simulink model "roadIntersection"  (R2017a)
settings: Solver=VariableStepAuto  StartTime=0  StopTime=40  MaxStep=0.05  RelTol=1e-3
model workspace (MAT data in the model file):
  MCOS : class17 (value not decoded)
  MCOS : class17 (value not decoded)
  MCOS : class17 (value not decoded)
  MCOS : class17 (value not decoded)
  MCOS : class17 (value not decoded)
  MCOS : class17 (value not decoded)
  MCOS : class17 (value not decoded)
  MCOS : class17 (value not decoded)
values from neighbouring files (symbols this model uses):
  D = getSimulinkBlockHandle('experiment/Orientation')    [configModel.m]
  m = rt.find('-isa','Simulink.BlockDiagram','-and','Name',mdl)    [configModel.m]
  MIN_SAFE_DIST = 1    [simulation.m]    (also in stateflowSim.m)
  V = getSimulinkBlockHandle('experiment/Velocity')    [configModel.m]
  WORLD_SIZE = 8    [simulation.m]    (also in stateflowSim.m)
  X = getSimulinkBlockHandle('experiment/Position')    [configModel.m]
undefined symbols (not defined in the file or in its folder): DrivingState, n, Stateflow
libraries: libraries x28
(part 2 of 2)

== stateflow chart roadIntersection/Conservative ==
  state Left
    en:
    [pf,df] = prepareLeft(this);
    S(this) = DrivingState.LeftTurn;
    TURN.data(1) = -1.5;
    send(TURN);
    state Normal
      state Clear
      state Check
      (default) -> Left.Normal.Clear
      Left.Normal.Clear -> Check : [isCloseToCheck(this) && ...
          | hasOncomingCar(this)]
          | {send(BRAKE);}
      Check -> Left.Normal.Clear : [~hasOncomingCar(this)]
          | {send(GAS);}
    state WAIT
    Left.Normal -> Left.WAIT : [detectPedestrian]
    Left.WAIT -> Left.Normal : [~hasPedestrian(this,...
        | MIN_SAFE_DIST,...
        | 0.5*MIN_SAFE_DIST)]
        | {send(GAS);}
    (default) -> Left.Normal
  note: Helper Funcs
  note: Left Turn
  note: Right Turn
  note: Perception
  state Right
    en:
    [pf,df] = prepareRight(this);
    TURN.data(1) = 0.5;
    send(TURN);
    S(this) = DrivingState.RightTurn;
    state Normal
    state WAIT
    Right.Normal -> Right.WAIT : [detectPedestrian]
    Right.WAIT -> Right.Normal : [~hasPedestrian(this,...
        | MIN_SAFE_DIST,...
        | 0.5*MIN_SAFE_DIST)]
        | {send(GAS);}
    (default) -> Right.Normal
  state Straight
    en:
    S(this) = DrivingState.Straight;
    state HasFrontCar
      en:
      idx = frontCarIndex(this);
      state FollowBehind
        en:
        [dxnorm, dvnorm] = frontCarInfo(this,idx);
        du:
        [dxnorm, dvnorm] = frontCarInfo(this,idx);
        state Safe
          en:
          if dvnorm < 0
          disp('BRAKE');
          BRAKE.data = ...
          [norm(V(:,idx));A_MAX];
          send(BRAKE);
          else
          disp('GAS');
          GAS.data = ...
          [norm(V(:,idx));A_MAX]
          send(GAS);
          end
        state Dangerous
        Straight.HasFrontCar.FollowBehind.Safe -> Straight.HasFrontCar.FollowBehind.Dangerous : [dxnorm < 1.6 * MIN_SAFE_DIST]
            | {BRAKE.data = ...
            | [0.5*norm(V(:,idx));A_MAX];
            | send(BRAKE);}
        Straight.HasFrontCar.FollowBehind.Dangerous -> Straight.HasFrontCar.FollowBehind.Safe : [dxnorm > 2*MIN_SAFE_DIST]
        (junction 192) -> Straight.HasFrontCar.FollowBehind.Dangerous : {BRAKE.data = ...
            | [0;A_MAX];
            | send(BRAKE);}
        (junction 185) -> Straight.HasFrontCar.FollowBehind.Safe [order 1] : [dxnorm > 2 * MIN_SAFE_DIST]
        (default) -> (junction 185)
        (junction 185) -> (junction 192) [order 2]
    state FreeDriving
    (default) -> Straight.HasFrontCar [order 1] : [hasFrontCar(this)]
    (default) -> (junction 218) [order 2]
    Straight.HasFrontCar -> (junction 218) : [frontCarHasLeft(this)]
    (junction 218) -> Straight.FreeDriving : {GAS.data = [V_MAX;A_MAX];
        | send(GAS);}
    Straight.FreeDriving -> Straight.HasFrontCar : [hasFrontCar(this)]
  state Start
    en:
    GAS.data=[0;0];
    BRAKE.data=[0;0];
    TURN.data=[0;0];
    BACK.data=[0;0];
  state res = detectPedestrian [function]
    (default) -> (junction 241) : {res = false;}
    (junction 241) -> (junction 252) [order 1] : PEDES
    (junction 252) -> (junction 254) : {TRASH.data = PEDES.data;
        | forward(PEDES,TRASH);}
    (junction 254) -> (junction 241) : {res = true;}
    (junction 241) -> (junction 243) [order 2]
  state WAIT
  state RoadIntersection
    state FreeDriving
      state Normal
        state Green
          en:
          GAS.data = [V_MAX;A_MAX];
          send(GAS);
        state Stop
        state RushToPass
          en:
          GAS.data=...
          [V_MAX;A_MAX];
          send(GAS);
        (default) -> RoadIntersection.FreeDriving.Normal.Green [order 1] : [isGreen(this)]
        RoadIntersection.FreeDriving.Normal.Green -> (junction 211) : [isYellow(this)]
        RoadIntersection.FreeDriving.Normal.Stop -> RoadIntersection.FreeDriving.Normal.Green : [isGreen(this)]
        (junction 211) -> RoadIntersection.FreeDriving.Normal.Stop [order 1] : [norm(V(:,this)) == 0]
        (default) -> (junction 211) [order 2]
        (junction 211) -> (junction 209) [order 2]
        (junction 209) -> RushToPass [order 2]
        (junction 209) -> RoadIntersection.FreeDriving.Normal.Stop [order 1] : [isStoppable(this,inter)]
            | {BRAKE.data = ...
            | [0;requiredBrake(this,inter)];
            | send(BRAKE);}
      state Right
        state Clear
          state Green
            en:
            if norm(V(:,this)) < 1
            GAS.data = [1;A_MAX];
            send(GAS);
            elseif norm(V(:,this)) > 1
            BRAKE.data = [1;A_MAX];
            send(BRAKE);
            end
          state Stop
            en:
            if norm(V(:,this)) > 0
            BRAKE.data = ...
            [0;requiredBrake(this,inter)];
            send(BRAKE);
            end
          (default) -> RoadIntersection.FreeDriving.Right.Clear.Green [order 1] : [isGreen(this)]
          RoadIntersection.FreeDriving.Right.Clear.Stop -> RoadIntersection.FreeDriving.Right.Clear.Green : [isGreen(this)]
          RoadIntersection.FreeDriving.Right.Clear.Green -> RoadIntersection.FreeDriving.Right.Clear.Stop : [isYellow(this)]
          (default) -> RoadIntersection.FreeDriving.Right.Clear.Stop [order 2]
        state Wait
          en:
          BRAKE.data = ...
          [0;requiredBrake(this,inter)];
          send(BRAKE);
        (default) -> RoadIntersection.FreeDriving.Right.Clear [order 2]
        Wait -> RoadIntersection.FreeDriving.Right.Clear : [~pedCrossAtRight(inter)]
        RoadIntersection.FreeDriving.Right.Clear -> Wait : [pedCrossAtRight(inter)]
        (default) -> Wait [order 1] : [pedCrossAtRight(inter)]
      (default) -> RoadIntersection.FreeDriving.Normal [order 1] : [decision ~= Decision.Right]
      (default) -> RoadIntersection.FreeDriving.Right [order 2]
    state HasFrontCar
      en:
      idx = frontCarIndex(this);
      front = closestObj(this,X(:,idx),inter);
      du:
      front = closestObj(this,X(:,idx),inter);
      state FollowBehind
        en:
        [dxnorm, dvnorm] = frontCarInfo(this,idx);
        du:
        [dxnorm, dvnorm] = frontCarInfo(this,idx);
        state Safe
          en:
          if dvnorm < 0
          BRAKE.data(1) = ...
          norm(V(:,idx));
          send(BRAKE);
          else
          GAS.data(1) = ...
          norm(V(:,idx));
          send(GAS);
          end
        state Dangerous
        RoadIntersection.HasFrontCar.FollowBehind.Safe -> RoadIntersection.HasFrontCar.FollowBehind.Dangerous : [dxnorm < 1.4*MIN_SAFE_DIST]
            | {BRAKE.data = ...
            | [0.5*norm(V(:,this));A_MAX];
            | send(BRAKE);}
        RoadIntersection.HasFrontCar.FollowBehind.Dangerous -> RoadIntersection.HasFrontCar.FollowBehind.Safe : [dxnorm > 1.5*MIN_SAFE_DIST]
        (junction 200) -> RoadIntersection.HasFrontCar.FollowBehind.Dangerous : {BRAKE.data = ...
            | [0;A_MAX];
            | send(BRAKE);}
        (junction 198) -> RoadIntersection.HasFrontCar.FollowBehind.Safe [order 1] : [dxnorm > 1.5*MIN_SAFE_DIST]
        (default) -> (junction 198)
        (junction 198) -> (junction 200) [order 2]
      state Stop
        en:
        if norm(V(:,this)) > 0
        BRAKE.data = ...
        [0;requiredBrake(this,front)];
        send(BRAKE);
        end
      (default) -> RoadIntersection.HasFrontCar.FollowBehind [order 1] : [isGreen(this)]
      (default) -> (junction 182) [order 2]
      RoadIntersection.HasFrontCar.FollowBehind -> (junction 182) : [isYellow(this)]
      (junction 182) -> RoadIntersection.HasFrontCar.Stop
      RoadIntersection.HasFrontCar.Stop -> RoadIntersection.HasFrontCar.FollowBehind : [isGreen(this)]
    (default) -> RoadIntersection.FreeDriving
    RoadIntersection.FreeDriving -> RoadIntersection.HasFrontCar : [hasFrontCar(this)]
    RoadIntersection.HasFrontCar -> RoadIntersection.FreeDriving : [frontCarHasLeft(this) ||...
        | isequal(front,inter)]
  Left -> (junction 317) : [finishTurn(this,pf)]
      | {send(BACK);
      | inter = ...
      | resumeFromLeft(this,df);}
  (junction 76) -> Left
  (junction 317) -> (junction 318)
  (junction 48) -> (junction 76) [order 2]
  (junction 48) -> Right [order 1] : [decision == Decision.Right]
  (junction 44) -> (junction 48) [order 2]
  Right -> Straight : [finishTurn(this,pf)]
      | {send(BACK);
      | inter = ...
      | resumeFromRight(this,df);}
  (default) -> Start
  (junction 318) -> Straight
  Start -> Straight
  (junction 44) -> Straight [order 1] : [decision == Decision.Straight]
  RoadIntersection -> (junction 44) [order 1] : [passStopLine(this)]
  Straight -> RoadIntersection : [isCloseToInter(this)]
  WAIT -> RoadIntersection : [~hasPedestrian(this,...
      | MIN_SAFE_DIST,...
      | 0.5*MIN_SAFE_DIST)]
  RoadIntersection -> WAIT [order 2] : [detectPedestrian]
  data: dxfr function_output; self function_input; index function_input; dvfr function_output; self function_input; res function_output; self function_input uint8 size=1; p function_output; d function_output; self function_input; res function_output; lSafeDist function_input; sSafeDist function_input; self function_input uint8 size=1; d function_input; newInter function_output; self function_input uint8 size=1; d function_input; newInter function_output; self function_input; res function_output; self function_input; p function_input; res function_output; self function_input uint8 size=1; p function_output; d function_output; res function_output; currInter function_input; self function_input; res function_output; self function_input; idx function_output; self function_input; res function_output; self function_input; res function_output; self function_input; obj1 function_input; res function_output; obj2 function_input; self function_input; res function_output; self function_input; pos function_input; res function_output; dxnorm local; dvnorm local; idx local; self function_input; pos function_input; res function_output; self function_input; res function_output; res function_output; self function_input; res function_output; dxnorm local; dvnorm local; idx local; front local; inter local =[0.5; -1]; X data_store_memory; V data_store_memory; D data_store_memory; this local uint8 size=1 =uint8(2); GAS output; BRAKE output; MIN_SAFE_DIST parameter; light data_store_memory; WORLD_SIZE parameter; decision local Enum: Decision =Decision.Right; TURN output; pf local; df local; BACK output; V_MAX constant double =2.5; A_MAX constant double =2.5; P data_store_memory; PEDES input; TRASH local size=2; S data_store_memory
  function [dxfr,dvfr] = frontCarInfo(self,index):
    | function [dxfr,dvfr] = frontCarInfo(self,index)
    |  
    | x = X(:,self);
    | v = V(:,self);
    | d = D(:,self);
    | 
    | xfront = X(:,index);
    | vfront = V(:,index);
    | 
    | range = 2 * WORLD_SIZE;
    | 
    | dxfr = mod((dot(xfront - x, d)+range), range);
    | dvfr = dot(vfront-v, d);
  function res = hasOncomingCar(self):
    | function res = hasOncomingCar(self)
    |  
    | res = true;
    | 
    | xself = X(:, self);
    | xall = X;
    | [~,indx]=ismember(xself', xall', 'rows');
    | xall(:,indx) = [100; 100];
    | 
    | xmin = 0;
    | xmax = 0;
    | ymin = 0;
    | ymax = 0;
    | 
    | if isequal(inter, [0.5; -1])
    |     % region 1
    |     xmin = -1;
    |     ymax = 2.5;
    | elseif isequal(inter, [1; 0.5])
    |     % region 2
    |     ymin = -1;
    |     xmin = -2.5;
    | elseif isequal(inter, [-0.5; 1])
    |     % region 3 
    |     xmax = 1;
    |     ymin = -2.5;
    | elseif isequal(inter, [-1; -0.5])
    |     % region 4
    |     xmax = 2.5;
    |     ymax = 1;
    | else
    |     error('checkOncomingLane error');
    | end
    | 
    | xall = xall(:, (xall(1,:) >= xmin));
    | if ~isempty(xall)
    |     xall = xall(:, (xall(1,:) <= xmax));
    | else
    |     res = false;
    |     return;
    | end
    | if ~isempty(xall)
    |     xall = xall(:, (xall(2,:) >= ymin));
    | else
    |     res = false;
    |     return;
    | end
    | if ~isempty(xall)
    |     xall = xall(:, (xall(2,:) <= ymax));
    | else
    |     res = false;
    |     return;
    | end
  function [p, d] = prepareRight(self):
    | function [p, d] = prepareRight(self)
    | 
    | d0 = D(:,self);
    | p = [0; 0];
    | d = [0; 0];
    | 
    | if isequal(d0, [1; 0])
    |     p = [-0.5; -1];
    |     d = [0; -1];
    | elseif isequal(d0, [-1; 0])
    |     p = [0.5; 1];
    |     d = [0; 1];
    | elseif isequal(d0, [0; 1])
    |     p = [1; -0.5];
    |     d = [1; 0];
    | elseif isequal(d0, [0; -1])
    |     p = [-1; 0.5];
    |     d = [-1; 0];
    | else
    |     error('Unknown orientation');
    | end
  function res = hasPedestrian(self, lSafeDist, sSafeDist):
    | function res = hasPedestrian(self, lSafeDist, sSafeDist)
    | 
    | if ~any(P ~= -1)
    |     res = false;
    |     return;
    | end
    | 
    | FARAWAY = 100;
    | 
    | pi = [-1 1 1 1; -1 -1 1 1];
    | dp = [2 0 -2 0; 0 2 0 -2];
    | 
    | dx_norm = ones(4, 1) * FARAWAY;
    | x = X(:,self);
    | d = D(:,self);
    | 
    | offset = 0;
    | if S(self) == DrivingState.RightTurn
    |     offset = 0.5236;
    | elseif S(self) == DrivingState.LeftTurn
    |     offset = -0.5236;
    |     lSafeDist = 1.5*lSafeDist;
    | end
    | 
    | for k=1:length(P)
    |     
    |     if P(k) ~= -1
    |         p = pi(:,k) + dp(:,k) * P(k); 
    |         dx = p - x;
    |         
    |         check = dot(dx, d); 
    |         if check > 0
    |             
    |             dx_theta = atan2(dx(2), dx(1));
    |             d_theta = atan2(d(2), d(1));
    |             delta = d_theta - dx_theta;
    |         
    |             if delta > 3.1416 
    |                 delta = delta - 6.2832;
    |             elseif delta < -3.1416
    |                 delta = delta + 6.2832;
    |             end
    |             dx_norm(k) = norm(dx);
    |             
    |             % check nomalized angle lower than 30 degree
    |             if abs(delta-offset) > 0.5236 && (dx_norm(k) >= sSafeDist)
    |                 dx_norm(k) = FARAWAY;
    |             end
    |         end
    |         
    | %         check = dot(dx, d);
    | %         if check > 0
    | %             dx_norm(k) = norm(dx);
    | %             theta = acos(check/dx_norm(k));
    | %             if rad2deg(theta) > 30 && (dx_norm(k) >= sSafeDist)
    | %                 dx_norm(k) = FARAWAY;
    | %             end
    | %         end
    |     end
    | end
    | 
    | res = any(dx_norm <= 1 * lSafeDist);
  function newInter = resumeFromLeft(self, d):
    | function newInter = resumeFromLeft(self, d)
    | 
    | x = X(:,self);
    | 
    | if isequal(d, [1; 0])
    |     x = [1; -0.5];
    |     newInter = [-1; -0.5];
    | elseif isequal(d, [-1; 0])
    |     x = [-1; 0.5];
    |     newInter = [1; 0.5];
    | elseif isequal(d, [0; 1])
    |     x = [0.5; 1];
    |     newInter = [0.5; -1];
    | elseif isequal(d, [0; -1])
    |     x = [-0.5; -1];
    |     newInter = [-0.5; 1];
    | else
    |     error('Unknown orientation');
    | end
    | 
    | v = V(:,self);
    | 
    | X(:,self) = x;
    | V(:,self) = d * norm(v);
    | D(:,self) = d;
  function newInter = resumeFromRight(self, d):
    | function newInter = resumeFromRight(self, d)
    | 
    | x = X(:,self);
    | 
    | if isequal(d, [0; -1])
    |     x = [-0.5; -1];
    |     newInter = [-0.5; 1];
    | elseif isequal(d, [0; 1])
    |     x = [0.5; 1];
    |     newInter = [-0.5; -1];
    | elseif isequal(d, [1; 0])
    |     x = [1; -0.5];
    |     newInter = [-1; -0.5];
    | elseif isequal(d, [-1; 0])
    |     x = [-1; 0.5];
    |     newInter = [1; 0.5];
    | else
    |     error('Unknown orientation');
    | end
    | 
    | v = V(:,self);
    | 
    | X(:,self) = x;
    | V(:,self) = d * norm(v);
    | D(:,self) = d;
  function res = passStopLine(self):
    | function res = passStopLine(self)
    | 
    | x = X(:,self);
    | d = D(:,self);
    | 
    | dx_norm = dot(inter - x, d);
    | res = (dx_norm <= 0);
  function res = finishTurn(self, p):
    | function res = finishTurn(self, p)
    | 
    | x = X(:,self);
    | res = norm(x - p) <= 0.1;
  function [p, d] = prepareLeft(self):
    | function [p, d] = prepareLeft(self)
    | 
    | d0 = D(:,self);
    | p = [0; 0];
    | d = [0; 0];
    | 
    | if isequal(d0, [1; 0])
    |     p = [0.5; 1];
    |     d = [0; 1];
    | elseif isequal(d0, [-1; 0])
    |     p = [-0.5; -1];
    |     d = [0; -1];
    | elseif isequal(d0, [0; 1])
    |     p = [-1; 0.5];
    |     d = [-1; 0];
    | elseif isequal(d0, [0; -1])
    |     p = [1; -0.5];
    |     d = [1; 0];
    | else
    |     error('Unknown orientation');
    | end
  function res = pedCrossAtRight(currInter):
    | function res = pedCrossAtRight(currInter)
    | 
    | res = false;
    | if isequal(currInter, [-1; -0.5])
    |     res = ((P(1) >= 0) && (P(1) <= 0.5));
    | elseif isequal(currInter, [0.5; -1])
    |     res = ((P(2) >= 0) && (P(2) <= 0.5));
    | elseif isequal(currInter, [1; 0.5])
    |     res = ((P(3) >= 0) && (P(3) <= 0.5));
    | elseif isequal(currInter, [-0.5; 1])
    |     res = ((P(4) >= 0) && (P(4) <= 0.5));
    | else
    |     error('Unrecognized currInter!');
    | end
  function res = isCloseToInter(self):
    | function res = isCloseToInter(self)
    | 
    | x = X(:,self);
    | d = D(:,self);
    | 
    | dist = dot(inter-x, d);
    | res = ((dist > 0) && (dist <= 2.5*MIN_SAFE_DIST));
  function idx = frontCarIndex(self):
    | function idx = frontCarIndex(self)
    | 
    | FARAWAY = 100;
    | RANGE = 2*WORLD_SIZE;
    | 
    | dx = zeros(size(X, 2), 1);
    | x = X(:,self);
    | v = V(:,self);
    | d = D(:,self);
    | 
    | for k=1:length(dx)
    |     dx(k) = dot(X(:,k) - x, d);
    |     dx(k) = mod((dx(k)+RANGE), RANGE);
    | end
    | 
    | % set zero dX to a large enough value
    | dx(dx == 0) = FARAWAY;
    | [~, idx] = min(dx);
    | idx = uint8(idx);
  function res = isCloseToCheck(self):
    | function res = isCloseToCheck(self)
    | 
    | res = (norm(X(:,self)) <= 0.25);
  function res = isGreen(self):
    | function res = isGreen(self)
    | 
    | d = D(:,self);
    | 
    | % compute the corresponding traffic light
    | horizon = (abs(d(1)) ~= 0);
    | vertical = (abs(d(2)) ~= 0);
    | 
    | res = false;
    | if uint8(light) == 3 && horizon
    |     % horizontal: green, vertical: red
    |     res = true;
    | elseif uint8(light) == 1 && vertical
    |     % horizontal: red, vertical: green
    |     res = true;
    | end
  function res = closestObj(self, obj1, obj2):
    | function res = closestObj(self, obj1, obj2)
    | 
    | if isequal(obj1, obj2)
    |     res = obj1;
    |     return;
    | end
    | 
    | RANGE = 2*WORLD_SIZE;
    | 
    | x = X(:,self);
    | d = D(:,self);
    | 
    | dX = zeros(2, 1);
    | dX(1) = mod(dot(obj1 - x, d) + RANGE, RANGE);
    | dX(2) = mod(dot(obj2 - x, d) + RANGE, RANGE);
    | 
    | [~, index] = min(dX);
    | if index == 1
    |     res = obj1;
    | else
    |     res = obj2;
    | end
  function res = isYellow(self):
    | function res = isYellow(self)
    | 
    | d = D(:,self);
    | 
    | % compute the corresponding traffic light
    | horizon = (abs(d(1)) ~= 0);
    | vertical = (abs(d(2)) ~= 0);
    | 
    | res = false;
    | if uint8(light) == 4 && horizon
    |     % horizontal: yellow, vertical: red
    |     res = true;
    | elseif uint8(light) == 2 && vertical
    |     % horizontal: red, vertical: yellow
    |     res = true;
    | end
  function res = requiredBrake(self,pos):
    | function res = requiredBrake(self,pos)
    | 
    | x = X(:,self);
    | v = V(:,self);
    | d = D(:,self);
    | 
    | % add safe distance
    | range = 2 * WORLD_SIZE;
    | diff = mod((dot(pos - x, d)+range),range);
    | dist = diff - MIN_SAFE_DIST;
    | 
    | % assert(dist >= 0);
    | if dist < 0
    |     res = A_MAX;
    |     return;
    | end
    | 
    | vnorm = norm(v);
    | 
    | % add a 0.05 factor to accomadate the asynchronous behaviour
    | res = 1.05 * vnorm*vnorm/2/dist;
  function res = isStoppable(self,pos):
    | function res = isStoppable(self,pos)
    | 
    | x = X(:,self);
    | v = V(:,self);
    | d = D(:,self);
    | 
    | range = 2 * WORLD_SIZE;
    | diff = mod((dot(pos - x, d)+range), range) ;
    | dist = diff - MIN_SAFE_DIST;
    | 
    | v_norm = norm(v);
    | brakeDist = v_norm*v_norm/2.0/A_MAX;
    | res = (brakeDist <= dist);
  function res = hasFrontCar(self):
    | function res = hasFrontCar(self)
    | 
    | % constants
    | THRES = 2.25 * MIN_SAFE_DIST;
    | FARAWAY = 100;
    | RANGE = 2 * WORLD_SIZE;
    | 
    | res = false;
    | 
    | % row of X: coordinate, col of X: num of cars
    | num = size(X, 2);
    | if num == 1
    |     return;
    | end
    | 
    | dx = zeros(num, 1);
    | x = X(:,self);
    | d = D(:,self);
    | car_size = [0.3; 0.4];
    | 
    | for k=1:length(dx)
    |     
    |     % compute difference
    |     xdelta = X(:,k) - x;
    |     
    |     % parallel and vertical distance
    |     delta_p = dot(xdelta, d);
    |     delta_v = norm(xdelta - (d * delta_p));
    |     
    |     % vertical distance is larger than car width
    |     if delta_v < car_size(1)
    |         dx(k) = delta_p;
    |     else
    |         dx(k) = FARAWAY;
    |     end
    |     
    |     % a rounded world
    |     dx(k) = mod((dx(k)+RANGE), RANGE);
    | end
    | 
    | % set zero dX to a large enough value
    | dx(dx == 0) = FARAWAY;
    | closest = min(dx);
    | res = closest <= THRES;
  function res = frontCarHasLeft(self):
    | function res = frontCarHasLeft(self)
    | 
    | % Constants 
    | THRES = 2.5 * MIN_SAFE_DIST;
    | FARAWAY = 100;
    | RANGE = 2 * WORLD_SIZE;
    | 
    | % if only one car in the environment return directly
    | res = true;
    | num = size(X, 1);
    | if num == 1
    |     return;
    | end
    | 
    | % get the closet car index and its distance
    | dx = zeros(num, 1);
    | x = X(:,self);
    | d = D(:,self);
    | car_size = [0.3; 0.4];
    | 
    | for k=1:length(dx)
    |     
    |     xdelta = X(:,k) - x;
    |     xdelta_p = dot(xdelta, d);                  % parallel component
    |     xdelta_v = norm(xdelta - (d * xdelta_p));   % vertical component
    |     
    |     % when the vertical component is larger than the car width
    |     if xdelta_v < car_size(1)
    |         dx(k) = xdelta_p;
    |     else
    |         dx(k) = FARAWAY;
    |     end
    |     
    |     % since we are in the round world, normalize the distance if the 
    |     % front car is behind us 
    |     % a rounded world
    |     dx(k) = mod((dx(k)+RANGE), RANGE);
    | end
    | 
    | % set the zero dx to a large enough value for convenience
    | dx(dx == 0) = FARAWAY;
    | closest = min(dx);
    | res = closest > THRES;

== stateflow chart roadIntersection/PedestrianDetector ==
  state Init
    en:
    PEDES1.data = [0;A_MAX];
    PEDES2.data = [0;A_MAX];
  state IDLE
  state DETECTED
    en:
    send(PEDES1);
    send(PEDES2);
  (default) -> Init
  Init -> IDLE
  DETECTED -> IDLE : [~hasPedestrian(this,...
      | MIN_SAFE_DIST,...
      | 0.5*MIN_SAFE_DIST)]
  IDLE -> DETECTED : [hasPedestrian(this,...
      | MIN_SAFE_DIST,...
      | 0.5*MIN_SAFE_DIST)]
  data: self function_input; res function_output; lSafeDist function_input; sSafeDist function_input; PEDES1 output; X data_store_memory; this local uint8 size=1 =uint8(2); P data_store_memory; D data_store_memory; MIN_SAFE_DIST parameter; PEDES2 output; A_MAX constant double =2.5; S data_store_memory
  function res = hasPedestrian(self, lSafeDist, sSafeDist):
    | function res = hasPedestrian(self, lSafeDist, sSafeDist)
    | 
    | if ~any(P ~= -1)
    |     res = false;
    |     return;
    | end
    | 
    | FARAWAY = 100;
    | 
    | pi = [-1 1 1 1; -1 -1 1 1];
    | dp = [2 0 -2 0; 0 2 0 -2];
    | 
    | dx_norm = ones(4, 1) * FARAWAY;
    | x = X(:,self);
    | d = D(:,self);
    | 
    | % angle offset
    | offset = 0;
    | if S(self) == DrivingState.RightTurn
    |     offset = 0.5236;
    | elseif S(self) == DrivingState.LeftTurn
    |     offset = -0.5236;
    |     lSafeDist = 1.5*lSafeDist; 
    | end
    | 
    | for k=1:length(P)
    |     
    |     if P(k) ~= -1
    |         p = pi(:,k) + dp(:,k) * P(k);
    |         dx = p - x;
    |         check = dot(dx, d);
    |         
    |         % the pedestrian is infront of the car
    |         if check > 0
    |             dx_theta = atan2(dx(2), dx(1));
    |             d_theta = atan2(d(2), d(1));
    |             delta = d_theta - dx_theta;
    |         
    |             % normalize the angle to 
    |             if delta > 3.1416 
    |                 delta = delta - 6.2832;
    |             elseif delta < -3.1416
    |                 delta = delta + 6.2832;
    |             end
    |             dx_norm(k) = norm(dx);            
    |             
    |             % check nomalized angle lower than 30 degree
    |             if abs(delta-offset) > 0.5236 && (dx_norm(k) >= sSafeDist)
    |                 dx_norm(k) = FARAWAY;
    |             end
    |         end
    |         
    | %         check = dot(dx, d);
    | %         if check > 0
    | %             dx_norm(k) = norm(dx);
    | %             theta = acos(check/dx_norm(k));
    | %             if rad2deg(theta) > 30 && (dx_norm(k) >= sSafeDist)
    | %                 dx_norm(k) = FARAWAY;
    | %             end
    | %         end
    |     end
    | end
    | 
    | res = any(dx_norm <= 1 * lSafeDist);

== stateflow chart roadIntersection/Decision ==
  state res = detectPedestrian [function]
    (default) -> (junction 241) : {res = false;}
    (junction 241) -> (junction 252) [order 1] : PEDES
    (junction 252) -> (junction 254) : {TRASH.data = PEDES.data;
        | forward(PEDES,TRASH);}
    (junction 254) -> (junction 241) : {res = true;}
    (junction 241) -> (junction 243) [order 2]
  state Start
    en:
    GAS.data=[0;0];
    BRAKE.data=[0;0];
    TURN.data=[0;0];
    BACK.data=[0;0];
  state Left
  state Straight
    state HasFrontCar
      en:
      idx = frontCarIndex(this);
      state FollowBehind
        en:
        [dxnorm, dvnorm] = frontCarInfo(this,idx);
        du:
        [dxnorm, dvnorm] = frontCarInfo(this,idx);
        state Safe
          en:
          if dvnorm < 0
          BRAKE.data(1) = ...
          norm(V(:,idx));
          send(BRAKE);
          else
          GAS.data(1) = ...
          norm(V(:,idx));
          send(GAS);
          end
        state Dangerous
        Straight.HasFrontCar.FollowBehind.Safe -> Straight.HasFrontCar.FollowBehind.Dangerous : [dxnorm < 1.4 * MIN_SAFE_DIST]
            | {BRAKE.data = ...
            | [0.5*norm(V(:,idx));A_MAX];
            | send(BRAKE);}
        Straight.HasFrontCar.FollowBehind.Dangerous -> Straight.HasFrontCar.FollowBehind.Safe : [dxnorm > 1.6*MIN_SAFE_DIST]
        (junction 192) -> Straight.HasFrontCar.FollowBehind.Dangerous : {BRAKE.data = ...
            | [0;A_MAX];
            | send(BRAKE);}
        (junction 185) -> Straight.HasFrontCar.FollowBehind.Safe [order 1] : [dxnorm > 1.5 * MIN_SAFE_DIST]
        (default) -> (junction 185)
        (junction 185) -> (junction 192) [order 2]
    state FreeDriving
    (default) -> Straight.HasFrontCar [order 1] : [hasFrontCar(this)]
    (default) -> (junction 218) [order 2]
    Straight.HasFrontCar -> (junction 218) : [frontCarHasLeft(this)]
    (junction 218) -> Straight.FreeDriving : {GAS.data = [V_MAX;A_MAX];
        | send(GAS);}
    Straight.FreeDriving -> Straight.HasFrontCar : [hasFrontCar(this)]
  state Right
    state Normal
    state WAIT
    Right.Normal -> Right.WAIT : [detectPedestrian]
    Right.WAIT -> Right.Normal : [~hasPedestrian(this)]
        | {send(GAS);}
    (default) -> Right.Normal
  state RoadIntersection
    state FreeDriving
      state Normal
        state Green
          en:
          GAS.data = [V_MAX;A_MAX];
          send(GAS);
        state Stop
        state RushToPass
          en:
          GAS.data=...
          [V_MAX;A_MAX];
          send(GAS);
        (default) -> Green [order 1] : [isGreen(this)]
        Green -> (junction 211) : [isYellow(this)]
        RoadIntersection.FreeDriving.Normal.Stop -> Green : [isGreen(this)]
        (junction 211) -> RoadIntersection.FreeDriving.Normal.Stop [order 1] : [norm(V(:,this)) == 0]
        (default) -> (junction 211) [order 2]
        (junction 211) -> (junction 209) [order 2]
        (junction 209) -> RushToPass [order 2]
        (junction 209) -> RoadIntersection.FreeDriving.Normal.Stop [order 1] : [isStoppable(this,inter)]
            | {BRAKE.data = ...
            | [0;reqBrake(this,inter)];
            | send(BRAKE);}
      (default) -> RoadIntersection.FreeDriving.Normal
    state HasFrontCar
      en:
      idx = frontCarIndex(this);
      front = closestObj(this,X(:,idx),inter);
      du:
      front = closestObj(this,X(:,idx),inter);
      state FollowBehind
        en:
        [dxnorm, dvnorm] = frontCarInfo(this,idx);
        du:
        [dxnorm, dvnorm] = frontCarInfo(this,idx);
        state Safe
          en:
          if dvnorm < 0
          BRAKE.data(1) = ...
          norm(V(:,idx));
          send(BRAKE);
          else
          GAS.data(1) = ...
          norm(V(:,idx));
          send(GAS);
          end
        state Dangerous
        RoadIntersection.HasFrontCar.FollowBehind.Safe -> RoadIntersection.HasFrontCar.FollowBehind.Dangerous : [dxnorm < 1.4*MIN_SAFE_DIST]
            | {BRAKE.data = ...
            | [0.5*norm(V(:,this));A_MAX];
            | send(BRAKE);}
        RoadIntersection.HasFrontCar.FollowBehind.Dangerous -> RoadIntersection.HasFrontCar.FollowBehind.Safe : [dxnorm > 1.5*MIN_SAFE_DIST]
        (junction 200) -> RoadIntersection.HasFrontCar.FollowBehind.Dangerous : {BRAKE.data = ...
            | [0;A_MAX];
            | send(BRAKE);}
        (junction 198) -> RoadIntersection.HasFrontCar.FollowBehind.Safe [order 1] : [dxnorm > 1.5*MIN_SAFE_DIST]
        (default) -> (junction 198)
        (junction 198) -> (junction 200) [order 2]
      state Stop
      (default) -> RoadIntersection.HasFrontCar.FollowBehind [order 1] : [isGreen(this)]
      (default) -> (junction 182) [order 2]
      RoadIntersection.HasFrontCar.FollowBehind -> (junction 182) : [isYellow(this)]
      (junction 182) -> RoadIntersection.HasFrontCar.Stop : {BRAKE.data = ...
          | [0;reqBrake(this,front)];
          | send(BRAKE);}
      RoadIntersection.HasFrontCar.Stop -> RoadIntersection.HasFrontCar.FollowBehind : [isGreen(this)]
    (default) -> RoadIntersection.FreeDriving
    RoadIntersection.FreeDriving -> RoadIntersection.HasFrontCar : [hasFrontCar(this)]
    RoadIntersection.HasFrontCar -> RoadIntersection.FreeDriving : [frontCarHasLeft(this)]
  state WAIT
  (default) -> Start
  (junction 76) -> Left : [decision == Decision.Left]
      | {[pf,df] = prepareLeft(this);
      | TURN.data(1) = -1.5;
      | send(TURN);}
  Left -> Straight : [finishTurn(this,pf)]
      | {send(BACK);
      | inter = ...
      | resumeFromLeft(this,df);}
  (junction 48) -> (junction 76) [order 2]
  Start -> Straight
  (junction 48) -> Right [order 1] : [decision == Decision.Right]
      | {[pf,df] = prepareRight(this);
      | TURN.data(1) = 0.5;
      | send(TURN);}
  (junction 44) -> (junction 48) [order 2]
  Right -> Straight : [finishTurn(this,pf)]
      | {send(BACK);
      | inter = ...
      | resumeFromRight(this,df);}
  (junction 44) -> Straight [order 1] : [decision == Decision.Straight]
  RoadIntersection -> (junction 44) [order 1] : [passStopLine(this)]
  Straight -> RoadIntersection : [isCloseTo(this,inter)]
  RoadIntersection -> WAIT [order 2] : [detectPedestrian]
  WAIT -> RoadIntersection : [~hasPedestrian(this)]
  data: res function_output; self function_input uint8 size=1; d function_input; newInter function_output; self function_input uint8 size=1; p function_output; d function_output; self function_input; res function_output; dxfr function_output; self function_input; index function_input; dvfr function_output; self function_input; res function_output; self function_input; res function_output; pos function_input; dxnorm local; dvnorm local; idx local; self function_input; res function_output; self function_input; res function_output; self function_input; pos function_input; res function_output; dxnorm local; dvnorm local; idx local; front local; self function_input uint8 size=1; d function_input; newInter function_output; self function_input uint8 size=1; p function_output; d function_output; self function_input; p function_input; res function_output; self function_input; pos function_input; res function_output; self function_input; res function_output; self function_input; res function_output; self function_input; obj1 function_input; res function_output; obj2 function_input; self function_input; idx function_output; inter local =[0.5; -1]; X data_store_memory; V data_store_memory; D data_store_memory; this local uint8 size=1 =uint8(2); GAS output; BRAKE output; MIN_SAFE_DIST parameter; light data_store_memory; WORLD_SIZE parameter; decision local Enum: Decision =Decision.Right; TURN output; pf local; df local; BACK output; V_MAX constant double =2.5; A_MAX constant double =2.5; P data_store_memory; PEDES input; TRASH local size=2
  function newInter = resumeFromLeft(self, d):
    | function newInter = resumeFromLeft(self, d)
    | 
    | x = X(:,self);
    | 
    | if isequal(d, [1; 0])
    |     x = [1; -0.5];
    |     newInter = [-1; -0.5];
    | elseif isequal(d, [-1; 0])
    |     x = [-1; 0.5];
    |     newInter = [1; 0.5];
    | elseif isequal(d, [0; 1])
    |     x = [0.5; 1];
    |     newInter = [0.5; -1];
    | elseif isequal(d, [0; -1])
    |     x = [-0.5; -1];
    |     newInter = [-0.5; 1];
    | else
    |     error('Unknown orientation');
    | end
    | 
    | v = V(:,self);
    | 
    | X(:,self) = x;
    | V(:,self) = d * norm(v);
    | D(:,self) = d;
  function [p, d] = prepareLeft(self):
    | function [p, d] = prepareLeft(self)
    | 
    | d0 = D(:,self);
    | p = [0; 0];
    | d = [0; 0];
    | 
    | if isequal(d0, [1; 0])
    |     p = [0.5; 1];
    |     d = [0; 1];
    | elseif isequal(d0, [-1; 0])
    |     p = [-0.5; -1];
    |     d = [0; -1];
    | elseif isequal(d0, [0; 1])
    |     p = [-1; 0.5];
    |     d = [-1; 0];
    | elseif isequal(d0, [0; -1])
    |     p = [1; -0.5];
    |     d = [1; 0];
    | else
    |     error('Unknown orientation');
    | end
  function res = hasPedestrian(self):
    | function res = hasPedestrian(self)
    | 
    | if ~any(P ~= -1)
    |     res = false;
    |     return;
    | end
    | 
    | FARAWAY = 100;
    | 
    | pi = [-1 1 1 -1; -1 -1 1 1];
    | dp = [2 0 -2 0; 0 2 0 -2];
    | 
    | dx_norm = ones(4, 1) * FARAWAY;
    | x = X(:,self);
    | d = D(:,self);
    | 
    | for k=1:length(P)
    |     
    |     if P(k) ~= -1
    |         p = pi(:,k) + dp(:,k) * P(k); 
    |         dx = p - x;
    |         check = dot(dx, d);
    |         if check > 0
    |             dx_norm(k) = norm(dx);
    |             theta = acos(check/dx_norm(k));
    |             if rad2deg(theta) > 15
    |                 dx_norm(k) = FARAWAY;
    |             end
    |         end
    |     end
    | end
    | 
    | res = any(dx_norm <= 1 * MIN_SAFE_DIST);
  function [dxfr,dvfr] = frontCarInfo(self,index):
    | function [dxfr,dvfr] = frontCarInfo(self,index)
    |  
    | x = X(:,self);
    | v = V(:,self);
    | d = D(:,self);
    | 
    | xfront = X(:,index);
    | vfront = V(:,index);
    | 
    | range = 2 * WORLD_SIZE;
    | 
    | dxfr = mod((dot(xfront - x, d)+range), range);
    | dvfr = dot(vfront-v, d);
  function res = passStopLine(self):
    | function res = passStopLine(self)
    | 
    | x = X(:,self);
    | d = D(:,self);
    | 
    | dx_norm = dot(inter - x, d);
    | res = (dx_norm <= 0);
  function res = isCloseTo(self,pos):
    | function res = isCloseTo(self,pos)
    | 
    | x = X(:,self);
    | d = D(:,self);
    | 
    | dist = dot(pos-x, d);
    | res = ((dist > 0) && (dist <= 2.5*MIN_SAFE_DIST));
  function res = isGreen(self):
    | function res = isGreen(self)
    | 
    | d = D(:,self);
    | 
    | % compute the corresponding traffic light
    | horizon = (abs(d(1)) ~= 0);
    | vertical = (abs(d(2)) ~= 0);
    | 
    | res = false;
    | if uint8(light) == 3 && horizon
    |     % horizontal: green, vertical: red
    |     res = true;
    | elseif uint8(light) == 1 && vertical
    |     % horizontal: red, vertical: green
    |     res = true;
    | end
  function res = isYellow(self):
    | function res = isYellow(self)
    | 
    | d = D(:,self);
    | 
    | % compute the corresponding traffic light
    | horizon = (abs(d(1)) ~= 0);
    | vertical = (abs(d(2)) ~= 0);
    | 
    | res = false;
    | if uint8(light) == 4 && horizon
    |     % horizontal: yellow, vertical: red
    |     res = true;
    | elseif uint8(light) == 2 && vertical
    |     % horizontal: red, vertical: yellow
    |     res = true;
    | end
  function res = reqBrake(self,pos):
    | function res = reqBrake(self,pos)
    | 
    | x = X(:,self);
    | v = V(:,self);
    | d = D(:,self);
    | 
    | % add safe distance
    | range = 2 * WORLD_SIZE;
    | diff = mod((dot(pos - x, d)+range),range);
    | dist = diff - MIN_SAFE_DIST;
    | 
    | % assert(dist >= 0);
    | 
    | vnorm = norm(v);
    | res = vnorm*vnorm/2/dist;
  function newInter = resumeFromRight(self, d):
    | function newInter = resumeFromRight(self, d)
    | 
    | x = X(:,self);
    | 
    | if isequal(d, [0; -1])
    |     x = [-0.5; -1];
    |     newInter = [-0.5; 1];
    | elseif isequal(d, [0; 1])
    |     x = [0.5; 1];
    |     newInter = [-0.5; -1];
    | elseif isequal(d, [1; 0])
    |     x = [1; -0.5];
    |     newInter = [-1; -0.5];
    | elseif isequal(d, [-1; 0])
    |     x = [-1; 0.5];
    |     newInter = [1; 0.5];
    | else
    |     error('Unknown orientation');
    | end
    | 
    | v = V(:,self);
    | 
    | X(:,self) = x;
    | V(:,self) = d * norm(v);
    | D(:,self) = d;
  function [p, d] = prepareRight(self):
    | function [p, d] = prepareRight(self)
    | 
    | d0 = D(:,self);
    | p = [0; 0];
    | d = [0; 0];
    | 
    | if isequal(d0, [1; 0])
    |     p = [-0.5; -1];
    |     d = [0; -1];
    | elseif isequal(d0, [-1; 0])
    |     p = [0.5; 1];
    |     d = [0; 1];
    | elseif isequal(d0, [0; 1])
    |     p = [1; -0.5];
    |     d = [1; 0];
    | elseif isequal(d0, [0; -1])
    |     p = [-1; 0.5];
    |     d = [-1; 0];
    | else
    |     error('Unknown orientation');
    | end
  function res = finishTurn(self, p):
    | function res = finishTurn(self, p)
    | 
    | x = X(:,self);
    | res = norm(x - p) <= 0.1;
  function res = isStoppable(self,pos):
    | function res = isStoppable(self,pos)
    | 
    | x = X(:,self);
    | v = V(:,self);
    | d = D(:,self);
    | 
    | range = 2 * WORLD_SIZE;
    | diff = mod((dot(pos - x, d)+range), range) ;
    | dist = diff - MIN_SAFE_DIST;
    | 
    | v_norm = norm(v);
    | brakeDist = v_norm*v_norm/2.0/A_MAX;
    | res = (brakeDist <= dist);
  function res = hasFrontCar(self):
    | function res = hasFrontCar(self)
    | 
    | % constants
    | THRES = 1.8 * MIN_SAFE_DIST;
    | FARAWAY = 100;
    | RANGE = 2 * WORLD_SIZE;
    | 
    | res = false;
    | 
    | % row of X: coordinate, col of X: num of cars
    | num = size(X, 2);
    | if num == 1
    |     return;
    | end
    | 
    | dx = zeros(num, 1);
    | x = X(:,self);
    | d = D(:,self);
    | car_size = [0.3; 0.4];
    | 
    | for k=1:length(dx)
    |     
    |     % compute difference
    |     xdelta = X(:,k) - x;
    |     
    |     % parallel and vertical distance
    |     delta_p = dot(xdelta, d);
    |     delta_v = norm(xdelta - (d * delta_p));
    |     
    |     % vertical distance is larger than car width
    |     if delta_v < car_size(1)
    |         dx(k) = delta_p;
    |     else
    |         dx(k) = FARAWAY;
    |     end
    |     
    |     % a rounded world
    |     dx(k) = mod((dx(k)+RANGE), RANGE);
    | end
    | 
    | % set zero dX to a large enough value
    | dx(dx == 0) = FARAWAY;
    | closest = min(dx);
    | res = closest <= THRES;
  function res = frontCarHasLeft(self):
    | function res = frontCarHasLeft(self)
    | 
    | % Constants 
    | THRES = 2 * MIN_SAFE_DIST;
    | FARAWAY = 100;
    | RANGE = 2 * WORLD_SIZE;
    | 
    | % if only one car in the environment return directly
    | res = true;
    | num = size(X, 1);
    | if num == 1
    |     return;
    | end
    | 
    | % get the closet car index and its distance
    | dx = zeros(num, 1);
    | x = X(:,self);
    | d = D(:,self);
    | car_size = [0.3; 0.4];
    | 
    | for k=1:length(dx)
    |     
    |     xdelta = X(:,k) - x;
    |     xdelta_p = dot(xdelta, d);                  % parallel component
    |     xdelta_v = norm(xdelta - (d * xdelta_p));   % vertical component
    |     
    |     % when the vertical component is larger than the car width
    |     if xdelta_v < car_size(1)
    |         dx(k) = xdelta_p;
    |     else
    |         dx(k) = FARAWAY;
    |     end
    |     
    |     % since we are in the round world, normalize the distance if the 
    |     % front car is behind us 
    |     % a rounded world
    |     dx(k) = mod((dx(k)+RANGE), RANGE);
    | end
    | 
    | % set the zero dx to a large enough value for convenience
    | dx(dx == 0) = FARAWAY;
    | closest = min(dx);
    | res = closest > THRES;
  function res = closestObj(self, obj1, obj2):
    | function res = closestObj(self, obj1, obj2)
    | 
    | if isequal(obj1, obj2)
    |     res = obj1;
    |     return;
    | end
    | 
    | RANGE = 2*WORLD_SIZE;
    | 
    | x = X(:,self);
    | d = D(:,self);
    | 
    | dX = zeros(2, 1);
    | dX(1) = mod(dot(obj1 - x, d) + RANGE, RANGE);
    | dX(2) = mod(dot(obj2 - x, d) + RANGE, RANGE);
    | 
    | [~, index] = min(dX);
    | if index == 1
    |     res = obj1;
    | else
    |     res = obj2;
    | end
  function idx = frontCarIndex(self):
    | function idx = frontCarIndex(self)
    | 
    | FARAWAY = 100;
    | RANGE = 2*WORLD_SIZE;
    | 
    | dx = zeros(size(X, 2), 1);
    | x = X(:,self);
    | v = V(:,self);
    | d = D(:,self);
    | 
    | for k=1:length(dx)
    |     dx(k) = dot(X(:,k) - x, d);
    |     dx(k) = mod((dx(k)+RANGE), RANGE);
    | end
    | 
    | % set zero dX to a large enough value
    | dx(dx == 0) = FARAWAY;
    | [~, idx] = min(dx);
    | idx = uint8(idx);
